simulink model "ConcentracaoDeA"  (R2019a)
settings: Solver=VariableStepAuto  StartTime=0.0  StopTime=10.0  RelTol=1e-3
settings Model: Creator=Usuario  LastModifiedBy=Usuario

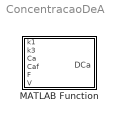
== system ConcentracaoDeA ==
  MATLAB Function : MATLAB Function  TreatAsAtomicUnit=on

== matlab function ConcentracaoDeA/MATLAB Function ==
  data: k1 input; DCa output; k3 input; Ca input; Caf input; F input; V input
function DCa = fcn(k1,k3,Ca,Caf,F,V)

DCa = -k1*Ca - k3*Ca^2 + (Caf -Ca)*F/V;
